simulink model "Motor_Controller"  (R2022a)
settings: Solver=FixedStepDiscrete  StartTime=0.0  StopTime=10.0  FixedStep=Tsi  RelTol=1e-3
values from neighbouring files (symbols this model uses):
  ID_MAP = -123.48613339558477 -123.48613339558477 -123.48613339558477 -123.48613339558477 -44.198759048598419 -53.055770135943519 -71.182249124603388 -83.754050470588808 -83.201735347031459 -88.439458490896953 -101.31743895897192 -109.70740328327217 -114.47442297164962 -116.44804085880824 -116.44444689073586 -115.21087408201925 -125.05741434421833 -119.17821915431119 -119.17821915431119 -119.17821915431119    [PMSM_plant_parameters.sldd]
  IQ_MAP = -339.52155191430609 -339.52155191430609 -339.52155191430609 -339.52155191430609 -298.63834091778995 -232.87622090578927 -192.99576989130705 -164.33367060179748 -138.47181888093323 -120.45650086696185 -110.27189121497848 -100.86088998300514 -91.979080238554033 -83.43921869931269 -75.095588141715126 -66.8406312898249 -66.136785837456742 -332.77622591535993 -332.77622591535993 -332.77622591535993 -33    [PMSM_plant_parameters.sldd]
  Ki_id = 710.3004    [ctrl_parameters.sldd]
  Ki_iq = 1061.5    [ctrl_parameters.sldd]
  Ki_omega = 200.0    [ctrl_parameters.sldd]
  Kp_id = 0.8779    [ctrl_parameters.sldd]
  Kp_iq = 1.0744    [ctrl_parameters.sldd]
  Kp_omega = 3.5    [ctrl_parameters.sldd]
  Ld = 0.00024368    [PMSM_plant_parameters.sldd]
  Lq = 0.00029758    [PMSM_plant_parameters.sldd]
  p = 8.0    [PMSM_plant_parameters.sldd]
  Pmax = 35000.0    [PMSM_plant_parameters.sldd]
  psim = 0.04366    [PMSM_plant_parameters.sldd]
  RPM_VECT = 0.0 500.0 1000.0 1500.0 2000.0 2500.0 3000.0 3500.0 4000.0 4500.0 5000.0 5500.0 6000.0 6500.0 7000.0 7500.0 8000.0    [PMSM_plant_parameters.sldd]
  Tmax = 205.0    [PMSM_plant_parameters.sldd]
  TQ_VECT = -205.0 -200.0 -195.0 -190.0 -185.0 -180.0 -175.0 -170.0 -165.0 -160.0 -155.0 -150.0 -145.0 -140.0 -135.0 -130.0 -125.0 -120.0 -115.0 -110.0 -105.0 -100.0 -95.0 -90.0 -85.0 -80.0 -75.0 -70.0 -65.0 -60.0 -55.0 -50.0 -45.0 -40.0 -35.0 -30.0 -25.0 -20.0 -15.0 -10.0 -5.0 0.0 5.0 10.0 15.0 20.0 25.0 30.0 35.0 40.0 45.0 50.0 55.0 60.0 65.0 70.0 75.0 80.0 85.0 90.0 95.0 100.0 105.0 110.0 115.0 120.0 125.0    [PMSM_plant_parameters.sldd]
  Tsi = 0.0001    [PMSM_system_data.sldd]
  Tso = 0.001    [PMSM_system_data.sldd]
  VDC_VECT = 275.0 300.0 325.0 350.0    [PMSM_plant_parameters.sldd]
  Vnom = 325.0    [PMSM_plant_parameters.sldd]
undefined symbols (not defined in the file or in its folder): denZC_id, denZC_iq, denZC_w, DiscIntNeverNeededParam, ee_sli_rtmsupport, gcbh, numZC_id, numZC_iq, numZC_w
libraries: simulink x8, eeTransforms x2
(part 1 of 2)
settings Model: DataDictionary=PMSM_system_data.sldd  Creator=tshintai  LastModifiedBy=tshintai
settings SolverCC: AlgebraicLoopSolver=TrustRegion
settings DataIOCC: SaveOutput=off  SignalLogging=off  DSMLogging=off  SaveTime=off  ReturnWorkspaceOutputs=off
settings OptimizationCC: DefaultParameterBehavior=Inlined  EnhancedBackFolding=on  PassReuseOutputArgsAs=Individual arguments  ZeroExternalMemoryAtStartup=off  ZeroInternalMemoryAtStartup=off  OptimizeBlockOrder=speed  DifferentSizesBufferReuse=on  OptimizationCustomize=off  EfficientTunableParamExpr=on
settings DebuggingCC: ParameterPrecisionLossMsg=none  ParameterTunabilityLossMsg=error  UnconnectedInputMsg=warning  UnconnectedOutputMsg=warning  UnconnectedLineMsg=warning  SFMachineParentedDataDiag=warning
settings SFSimCC: MATLABDynamicMemAlloc=off
settings RTWCC: SystemTargetFile=ert.tlc  GenCodeOnly=on  TemplateMakefile=ert_default_tmf  GenerateReport=on  IncludeHyperlinkInReport=on  LaunchReport=on  GenerateTraceInfo=on  GenerateTraceReport=on  GenerateTraceReportSl=on  GenerateTraceReportSf=on  GenerateTraceReportEml=on  GenerateCodeMetricsReport=on  DLArmComputeVersion=19.05
settings CodeAppCC: ForceParamTrailComments=on  IgnoreCustomStorageClasses=off  OperatorAnnotations=on  SimulinkDataObjDesc=on  SFDataObjDesc=on  InsertBlockDesc=on
settings ERTTargetCC: TargetLangStandard=C99 (ISO)  GenerateSampleERTMain=on  InlinedParameterPlacement=NonHierarchical  ERTCustomFileTemplate=example_file_process.tlc  EnableUserReplacementTypes=on

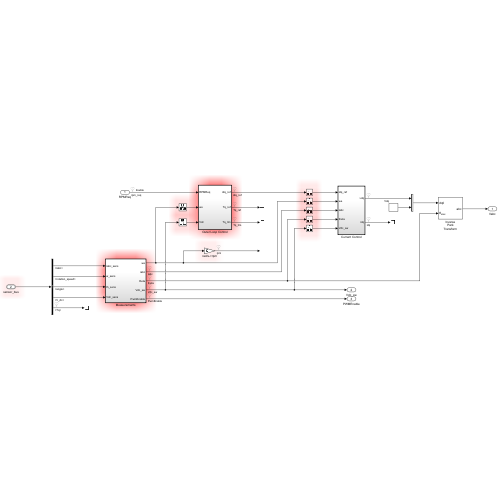
[thumbnail: Simulink's stored preview of the top-level diagram]
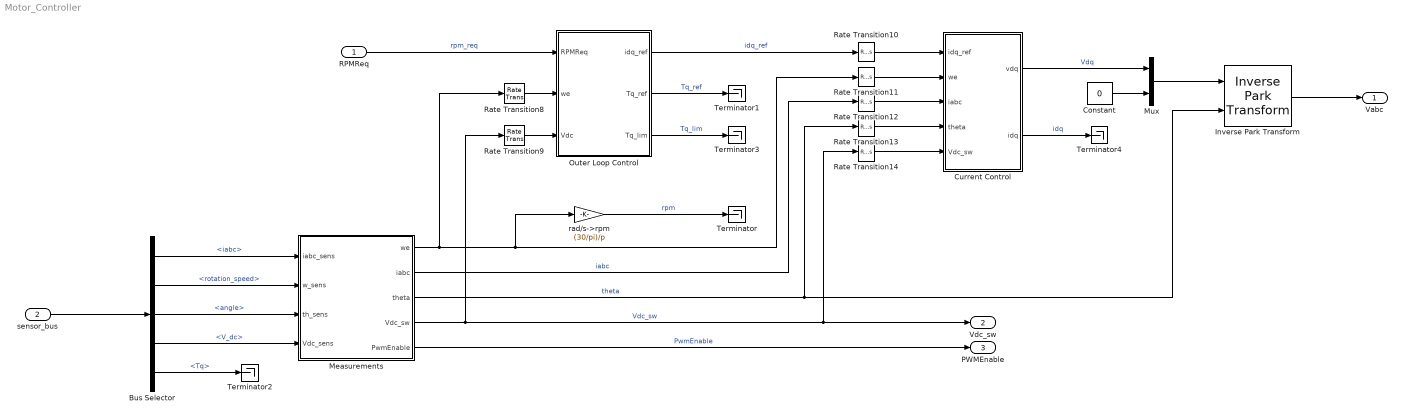
== system Motor_Controller ==
  RPMReq : Inport  OutDataTypeStr=double  PortDimensions=1
  sensor_bus : Inport  Port=2  OutDataTypeStr=Bus: sensor_bus
  Bus Selector : BusSelector  OutputSignals=iabc,rotation_speed,angle,V_dc,Tq
  Constant : Constant  Value=0  OutDataTypeStr=single  SampleTime=-1
  Current Control : Subsystem  TreatAsAtomicUnit=on  SystemSampleTime=1e-4
  Inverse Park Transform : eeTransforms/Inverse Park Transform  AxisAlignment=Q-axis  PowerInvariant=off
  Measurements : Subsystem  TreatAsAtomicUnit=on  SystemSampleTime=Tsi
  Mux : Mux  Inputs=2
  Outer Loop Control : Subsystem  TreatAsAtomicUnit=on  SystemSampleTime=Tso
  Rate Transition{10..14} (5 alike) : RateTransition  OutPortSampleTime=Tsi
  Rate Transition8 : RateTransition  OutPortSampleTime=Tso
  Rate Transition9 : RateTransition  OutPortSampleTime=Tso
  Terminator{,1..4} (5 alike) : Terminator
  rad/s->rpm : Gain  Gain=(30/pi)/p
  Vabc : Outport  VectorParamsAs1DForOutWhenUnconnected=off
  Vdc_sw : Outport  Port=2
  PWMEnable : Outport  Port=3
  wires:
  Rate Transition12/1 -> Current Control/3(iabc)
  Rate Transition13/1 -> Current Control/4(theta)
  Rate Transition14/1 -> Current Control/5(Vdc_sw)
  Bus Selector/1 -> Measurements/1(iabc_sens)  "<iabc>"
  RPMReq/1 -> Outer Loop Control/1(RPMReq)  "rpm_req"
  Bus Selector/2 -> Measurements/2(w_sens)  "<rotation_speed>"
  Mux/1 -> Inverse Park Transform/1
  Measurements/1(we) -> Rate Transition11/1, rad/s->rpm/1, Rate Transition8/1
  Measurements/2(iabc) -> Rate Transition12/1  "iabc"
  Outer Loop Control/1(idq_ref) -> Rate Transition10/1  "idq_ref"
  Current Control/1(vdq) -> Mux/1  "Vdq"
  Current Control/2(idq) -> Terminator4/1  "idq"
  Bus Selector/5 -> Terminator2/1  "<Tq>"
  Measurements/5(PwmEnable) -> PWMEnable/1  "PwmEnable"
  Bus Selector/3 -> Measurements/3(th_sens)  "<angle>"
  Constant/1 -> Mux/2
  Outer Loop Control/3(Tq_lim) -> Terminator3/1  "Tq_lim"
  Rate Transition8/1 -> Outer Loop Control/2(we)
  sensor_bus/1 -> Bus Selector/1
  Bus Selector/4 -> Measurements/4(Vdc_sens)  "<V_dc>"
  Rate Transition10/1 -> Current Control/1(idq_ref)
  Measurements/4(Vdc_sw) -> Vdc_sw/1, Rate Transition14/1, Rate Transition9/1  "Vdc_sw"
  Rate Transition9/1 -> Outer Loop Control/3(Vdc)
  Rate Transition11/1 -> Current Control/2(we)
  Inverse Park Transform/1 -> Vabc/1
  Measurements/3(theta) -> Rate Transition13/1, Inverse Park Transform/2  "theta"
  Outer Loop Control/2(Tq_ref) -> Terminator1/1  "Tq_ref"
  rad/s->rpm/1 -> Terminator/1  "rpm"

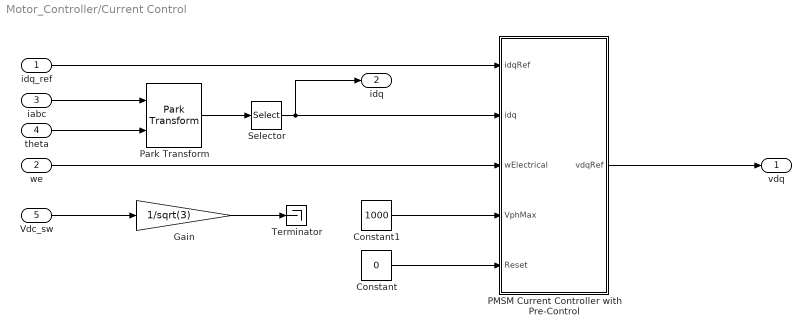
== system Motor_Controller/Current Control ==
  idq_ref : Inport
  we : Inport  Port=2
  iabc : Inport  Port=3
  theta : Inport  Port=4
  Vdc_sw : Inport  Port=5
  Constant : Constant  Value=0  OutDataTypeStr=boolean  SampleTime=-1
  Constant1 : Constant  Value=1000
  Gain : Gain  Gain=1/sqrt(3)
  PMSM Current Controller with Pre-Control : Subsystem  LoadFcn=ee_sli_rtmsupport( 'loadfcn', gcbh );  mask(PMSM Current Controller with Pre-Control){Kp_id=Kp_id, Ki_id=Ki_id, Kaw_id=1, Kp_iq=Kp_iq, Ki_iq=Ki_iq, Kaw_iq=1, Ts=-1, Tsd=Tsi, AxisPrio=Q-axis, ActZC=on, ActFF=on, idVect=[-200, 0, 200], iqVect=[-200, 0, 200], LdMatrix=Ld * ones(3, 3), LqMatrix=Lq * ones(3, 3), psimMatrix=psim * ones(3, 3)}
      mask prompts: Kp_id "physmod:ee:library:comments:control:eePmsmCurrentController:DaxisCurrentProportionalGain_MP"; Ki_id "physmod:ee:library:comments:control:eePmsmCurrentController:DaxisCurrentIntegralGain_MP"; Kaw_id "physmod:ee:library:comments:control:eePmsmCurrentController:DaxisCurrentAntiwindupGain_MP"; Kp_iq "physmod:ee:library:comments:control:eePmsmCurrentController:QaxisCurrentProportionalGain_MP"; Ki_iq "physmod:ee:library:comments:control:eePmsmCurrentController:QaxisCurrentIntegralGain_MP"; Kaw_iq "physmod:ee:library:comments:control:eePmsmCurrentController:QaxisCurrentAntiwindupGain_MP"; Ts "physmod:ee:library:comments:control:eePmsmCurrentController:SampleTime1ForInherited_MP"; Tsd "physmod:ee:library:comments:control:eePmsmCurrentController:DiscretizationSampleTime_MP"; AxisPrio "physmod:ee:library:comments:control:eePmsmCurrentController:AxisPrioritization_MP"; ActZC "physmod:ee:library:comments:control:eePmsmCurrentController:EnableZeroCancellation_MP"; ActFF "physmod:ee:library:comments:control:eePmsmCurrentController:EnablePrecontrolVoltage_MP"; idVect "physmod:ee:library:comments:control:eePmsmCurrentController:DaxisCurrentVectorIdA_MP"; iqVect "physmod:ee:library:comments:control:eePmsmCurrentController:QaxisCurrentVectorIqA_MP"; LdMatrix "physmod:ee:library:comments:control:eePmsmCurrentController:LdMatrixLdidiqH_MP"; LqMatrix "physmod:ee:library:comments:control:eePmsmCurrentController:LqMatrixLqidiqH_MP"; psimMatrix "physmod:ee:library:comments:control:eePmsmCurrentController:PermanentMagnetFluxLinkageMatrixPMidiqWb_MP"
      mask help: physmod:ee:library:comments:control:eePmsmCurrentController:PMSMCurrentControllerWithPreControl_MD
      mask init:
      | [Tsd, numZC_id, denZC_id, numZC_iq, denZC_iq] = ee.mask.initializePmsmCurrentController(ActZC,Ts,Tsd,Kp_id,Ki_id,Kp_iq,Ki_iq);
      | 
      | if length(idVect) < 2            
      | 	error(message('physmod:simscape:compiler:patterns:checks:LengthGreaterThanOrEqual',getString(message('physmod:ee:library:comments:control:eePmsmCurrentController:DaxisCurrentVectorIdA_MP')), '2'));            
      | end
      | if ~all(diff(idVect) > 0)            
      | 	error(message('physmod:simscape:compiler:patterns:checks:StrictlyAscendingVec',getString(message('physmod:ee:library:comments:control:eePmsmCurrentController:DaxisCurrentVectorIdA_MP'))));            
      | end
      | if length(iqVect) < 2            
      | 	error(message('physmod:simscape:compiler:patterns:checks:LengthGreaterThanOrEqual',getString(message('physmod:ee:library:comments:control:eePmsmCurrentController:QaxisCurrentVectorIqA_MP')), '2'));            
      | end
      | if ~all(diff(iqVect) > 0)            
      | 	error(message('physmod:simscape:compiler:patterns:checks:StrictlyAscendingVec',getString(message('physmod:ee:library:comments:control:eePmsmCurrentController:QaxisCurrentVectorIqA_MP'))));            
      | end
      | if ~all(size(LdMatrix) == [length(idVect), length(iqVect)])            
      | 	error(message('physmod:simscape:compiler:patterns:checks:Size2DEqual',getString(message('physmod:ee:library:comments:control:eePmsmCurrentController:LdMatrixLdidiqH_MP')), getString(message('physmod:ee:library:comments:control:eePmsmCurrentController:DaxisCurrentVectorIdA_MP')), getString(message('physmod:ee:library:comments:control:eePmsmCurrentController:QaxisCurrentVectorIqA_MP'))));            
      | end
      | if ~all(size(LqMatrix) == [length(idVect), length(iqVect)])            
      | 	error(message('physmod:simscape:compiler:patterns:checks:Size2DEqual',getString(message('physmod:ee:library:comments:control:eePmsmCurrentController:LqMatrixLqidiqH_MP')), getString(message('physmod:ee:library:comments:control:eePmsmCurrentController:DaxisCurrentVectorIdA_MP')), getString(message('physmod:ee:library:comments:control:eePmsmCurrentController:QaxisCurrentVectorIqA_MP'))));            
      | end
      | if ~all(size(psimMatrix) == [length(idVect), length(iqVect)])            
      | 	error(message('physmod:simscape:compiler:patterns:checks:Size2DEqual',getString(message('physmod:ee:library:comments:control:eePmsmCurrentController:PermanentMagnetFluxLinkageMatrixPMidiqWb_MP')), getString(message('physmod:ee:library:comments:control:eePmsmCurrentController:DaxisCurrentVectorIdA_MP')), getString(message('physmod:ee:library:comments:control:eePmsmCurrentController:QaxisCurrentVectorIqA_MP'))));            
      | end
      settings: CopyFcn=ee_sli_rtmsupport( 'copyfcn', gcbh );  DeleteFcn=ee_sli_rtmsupport( 'deletefcn', gcbh );  ModelCloseFcn=ee_sli_rtmsupport( 'modelclosefcn', gcbh );  PostSaveFcn=ee_sli_rtmsupport( 'postsavefcn', gcbh );  PreCopyFcn=ee_sli_rtmsupport( 'precopyfcn', gcbh );  OpenFcn=ee_sli_rtmsupport( 'openfcn', gcbh );  CloseFcn=ee_sli_rtmsupport( 'closefcn', gcbh );  PreDeleteFcn=ee_sli_rtmsupport( 'predeletefcn', gcbh );
      mask Help: web(nesl_help(gcbh))
      mask Callback Ts: ee.mask.callbackZeroCancellation(gcb);
      mask TypeOptions AxisPrio: d-q Voltage Limiter/AxisPrio
      mask Callback ActZC: ee.mask.callbackZeroCancellation(gcb);
      mask DialogControl Container3 Prompt: physmod:ee:library:comments:control:eePmsmCurrentController:tab_ControlParameters
      mask DialogControl Kp_id Prompt: D 軸電流の比例ゲイン
      mask DialogControl Ki_id Prompt: D 軸電流の積分ゲイン
      mask DialogControl Kaw_id Prompt: D 軸電流のアンチワインドアップ ゲイン
      mask DialogControl Kp_iq Prompt: Q 軸電流の比例ゲイン
      mask DialogControl Ki_iq Prompt: Q 軸電流の積分ゲイン
      mask DialogControl Kaw_iq Prompt: Q 軸電流のアンチワインドアップ ゲイン
      mask DialogControl Ts Prompt: サンプル時間 (継承は -1)
      mask DialogControl Tsd Prompt: 離散化サンプル時間
      mask DialogControl AxisPrio Prompt: 軸の優先順位付け
      mask DialogControl ActZC Prompt: 零点相殺を有効にする
      mask DialogControl ActFF Prompt: プリ制御電圧を有効にする
      mask DialogControl Container4 Prompt: physmod:ee:library:comments:control:eePmsmCurrentController:tab_PreControlParameters
      mask DialogControl idVect Prompt: D 軸電流ベクトル、id (A)
      mask DialogControl iqVect Prompt: Q 軸電流ベクトル、iq (A)
      mask DialogControl LdMatrix Prompt: Ld 行列、Ld(id,iq)、(H)
      mask DialogControl LqMatrix Prompt: Lq 行列、Lq(id,iq)、(H)
      mask DialogControl psimMatrix Prompt: 永久磁石の鎖交磁束の行列、PM(id,iq)、(Wb)
  Park Transform : eeTransforms/Park Transform  AxisAlignment=Q-axis  PowerInvariant=off
  Selector : Selector  InputPortWidth=3  IndexOptions=Index vector (dialog)  Indices=[1 2]  OutputSizes=1
  Terminator : Terminator
  vdq : Outport  VectorParamsAs1DForOutWhenUnconnected=off
  idq : Outport  Port=2  VectorParamsAs1DForOutWhenUnconnected=off
  wires:
  Vdc_sw/1 -> Gain/1
  iabc/1 -> Park Transform/1
  we/1 -> PMSM Current Controller with Pre-Control/3(wElectrical)
  theta/1 -> Park Transform/2
  PMSM Current Controller with Pre-Control/1(vdqRef) -> vdq/1
  idq_ref/1 -> PMSM Current Controller with Pre-Control/1(idqRef)
  Constant/1 -> PMSM Current Controller with Pre-Control/5(Reset)
  Selector/1 -> idq/1, PMSM Current Controller with Pre-Control/2(idq)
  Park Transform/1 -> Selector/1
  Gain/1 -> Terminator/1
  Constant1/1 -> PMSM Current Controller with Pre-Control/4(VphMax)

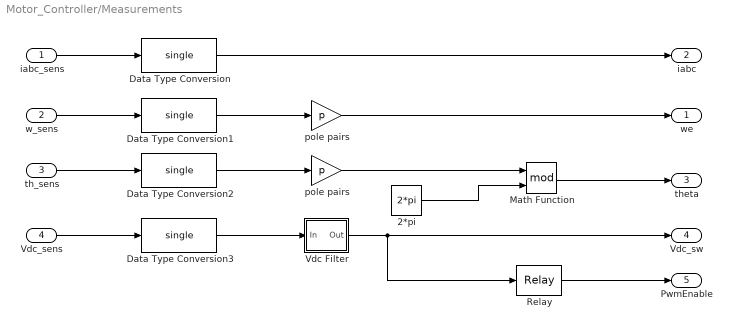
== system Motor_Controller/Measurements ==
  iabc_sens : Inport
  w_sens : Inport  Port=2
  th_sens : Inport  Port=3
  Vdc_sens : Inport  Port=4
  2*pi : Constant  Value=2*pi  OutDataTypeStr=single  SampleTime=-1
  Data Type Conversion{,1..3} (4 alike) : DataTypeConversion  OutDataTypeStr=single  SaturateOnIntegerOverflow=off  RndMeth=Floor
  Math Function : Math  Operator=mod  SignedPower=on
  Relay : Relay  OnSwitchValue=VDC_VECT(1)  OffSwitchValue=0.5*VDC_VECT(1)  OutDataTypeStr=boolean
  Vdc Filter : Subsystem  mask(Discrete first-order filter (Low-pass)){T=0.005, Ts=1e-4}
      mask prompts: T "Time constant (s):"; Ts "Sample time (s):"
      mask help: This block implements a discrete low-pass filter. To calculate the coefficients, the block discretises a continuous low-pass filter using the Tustin method.
      mask init:
      | num = [ Ts/(2*T + Ts), Ts/(2*T + Ts)];
      | den = [ 1, -(2*T - Ts)/(2*T + Ts)];
  pole pairs : Gain  Gain=p
  "pole pairs " : Gain  Gain=p
  we : Outport  VectorParamsAs1DForOutWhenUnconnected=off
  iabc : Outport  Port=2  VectorParamsAs1DForOutWhenUnconnected=off
  theta : Outport  Port=3  VectorParamsAs1DForOutWhenUnconnected=off
  Vdc_sw : Outport  Port=4  VectorParamsAs1DForOutWhenUnconnected=off
  PwmEnable : Outport  Port=5  VectorParamsAs1DForOutWhenUnconnected=off
  wires:
  pole pairs/1 -> we/1
  Vdc_sens/1 -> Data Type Conversion3/1
  th_sens/1 -> Data Type Conversion2/1
  w_sens/1 -> Data Type Conversion1/1
  iabc_sens/1 -> Data Type Conversion/1
  "pole pairs "/1 -> Math Function/1
  2*pi/1 -> Math Function/2
  Math Function/1 -> theta/1
  Relay/1 -> PwmEnable/1
  Vdc Filter/1(Out) -> Relay/1, Vdc_sw/1
  Data Type Conversion/1 -> iabc/1
  Data Type Conversion1/1 -> pole pairs/1
  Data Type Conversion2/1 -> "pole pairs "/1
  Data Type Conversion3/1 -> Vdc Filter/1(In)

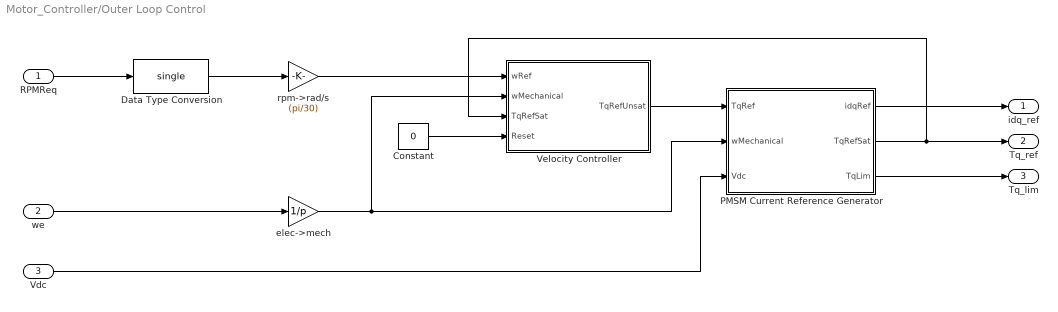
== system Motor_Controller/Outer Loop Control ==
  RPMReq : Inport
  we : Inport  Port=2
  Vdc : Inport  Port=3
  Constant : Constant  Value=0  OutDataTypeStr=boolean  SampleTime=-1
  Data Type Conversion : DataTypeConversion  OutDataTypeStr=single  SaturateOnIntegerOverflow=off  RndMeth=Floor
  PMSM Current Reference Generator : Subsystem  LoadFcn=ee_sli_rtmsupport( 'loadfcn', gcbh );  mask(PMSM Current Reference Generator){Vnom=Vnom, Pmax=Pmax, Tmax=Tmax, Ts=-1, RefType=Lookup-table based, rpmVec=RPM_VECT, TqVec=TQ_VECT, VdcVec=VDC_VECT, PWMMode=SVM: space vector modulation, ModFactor=1, idMatrix=ID_MAP, iqMatrix=IQ_MAP, p=8, psim=0.04, Ld=0.00024, Lq=0.00029, Rs=0.01, RefExpEnable=0}
      mask prompts: Vnom "physmod:ee:library:comments:control:eePmsmCurrentReferenceGen:NominalDclinkVoltageV_MP"; Pmax "physmod:ee:library:comments:control:eePmsmCurrentReferenceGen:MaximumPowerW_MP"; Tmax "physmod:ee:library:comments:control:eePmsmCurrentReferenceGen:MaximumTorqueNm_MP"; Ts "physmod:ee:library:comments:control:eePmsmCurrentReferenceGen:SampleTime1ForInherited_MP"; RefType "physmod:ee:library:comments:control:eePmsmCurrentReferenceGen:CurrentReferences_MP"; rpmVec "physmod:ee:library:comments:control:eePmsmCurrentReferenceGen:MechanicalSpeedVectorWMechanicalrpm_MP"; TqVec "physmod:ee:library:comments:control:eePmsmCurrentReferenceGen:TorqueReferenceVectorTqRefNm_MP"; VdcVec "physmod:ee:library:comments:control:eePmsmCurrentReferenceGen:DClinkVoltageVectorVdcV_MP"; PWMMode "physmod:ee:library:comments:control:eePmsmCurrentReferenceGen:PWMMethod_MP"; ModFactor "physmod:ee:library:comments:control:eePmsmCurrentReferenceGen:ModulationFactor_MP"; idMatrix "physmod:ee:library:comments:control:eePmsmCurrentReferenceGen:DaxisCurrentReferenceMatrixIdwMechanicalTqRefVdcA_MP"; iqMatrix "physmod:ee:library:comments:control:eePmsmCurrentReferenceGen:QaxisCurrentReferenceMatrixIqwMechanicalTqRefVdcA_MP"; p "physmod:ee:library:comments:control:eePmsmCurrentReferenceGen:NumberOfRotorPolePairs_MP"; psim "physmod:ee:library:comments:control:eePmsmCurrentReferenceGen:PermanentMagnetFluxLinkageWb_MP"; Ld "physmod:ee:library:comments:control:eePmsmCurrentReferenceGen:DaxisInductanceH_MP"; Lq "physmod:ee:library:comments:control:eePmsmCurrentReferenceGen:QaxisInductanceH_MP"; Rs "physmod:ee:library:comments:control:eePmsmCurrentReferenceGen:StatorResistanceOhm_MP"; RefExpEnable "physmod:ee:library:comments:control:eePmsmCurrentReferenceGen:ExportCurrentReferences_MP"
      mask help: physmod:ee:library:comments:control:eePmsmCurrentReferenceGen:PMSMCurrentReferenceGenerator_MD
      mask init:
      | if Vnom <= 0            
      |     error(message('physmod:simscape:compiler:patterns:checks:GreaterThanZero',getString(message('physmod:ee:library:comments:control:eePmsmCurrentReferenceGen:NominalDclinkVoltageV_MP'))));            
      | end
      | if Pmax <= 0            
      |     error(message('physmod:simscape:compiler:patterns:checks:GreaterThanZero',getString(message('physmod:ee:library:comments:control:eePmsmCurrentReferenceGen:MaximumPowerW_MP'))));            
      | end
      | if Tmax <= 0            
      |     error(message('physmod:simscape:compiler:patterns:checks:GreaterThanZero',getString(message('physmod:ee:library:comments:control:eePmsmCurrentReferenceGen:MaximumTorqueNm_MP'))));            
      | end
      | switch RefType
      |     case 'Zero d-axis control'
      |         EnableZDAC = 1;
      |         rpmVec = [0, 3000];
      |         TqVec  = [-100, 0, 100];
      |         VdcVec = [300, 350];
      |         idMatrix = zeros(2,3,2);
      |         iqMatrix = zeros(2,3,2);
      |     case 'Lookup-table based'
      |         EnableZDAC = 0;
      |         if length(rpmVec) < 2            
      |             error(message('physmod:simscape:compiler:patterns:checks:LengthGreaterThanOrEqual',getString(message('physmod:ee:library:comments:control:eePmsmCurrentReferenceGen:MechanicalSpeedVectorWMechanicalrpm_MP')), '2'));            
      |         end
      |         if ~all(diff(rpmVec) > 0)            
      |             error(message('physmod:simscape:compiler:patterns:checks:StrictlyAscendingVec',getString(message('physmod:ee:library:comments:control:eePmsmCurrentReferenceGen:MechanicalSpeedVectorWMechanicalrpm_MP'))));            
      |         end
      |         if length(TqVec) < 2            
      |             error(message('physmod:simscape:compiler:patterns:checks:LengthGreaterThanOrEqual',getString(message('physmod:ee:library:comments:control:eePmsmCurrentReferenceGen:TorqueReferenceVectorTqRefNm_MP')), '2'));            
      |         end
      |         if ~all(diff(TqVec) > 0)            
      |             error(message('physmod:simscape:compiler:patterns:checks:StrictlyAscendingVec',getString(message('physmod:ee:library:comments:control:eePmsmCurrentReferenceGen:TorqueReferenceVectorTqRefNm_MP'))));            
      |         end
      |         if length(VdcVec) < 2            
      |             error(message('physmod:simscape:compiler:patterns:checks:LengthGreaterThanOrEqual',getString(message('physmod:ee:library:comments:control:eePmsmCurrentReferenceGen:DClinkVoltageVectorVdcV_MP')), '2'));            
      |         end
      |         if ~all(diff(VdcVec) > 0)            
      |             error(message('physmod:simscape:compiler:patterns:checks:StrictlyAscendingVec',getString(message('physmod:ee:library:comments:control:eePmsmCurrentReferenceGen:DClinkVoltageVectorVdcV_MP'))));            
      |         end
      |         if ~all(size(idMatrix) == [length(rpmVec), length(TqVec), length(VdcVec)])            
      |             error(message('physmod:simscape:compiler:patterns:checks:Size3DEqual',getString(message('physmod:ee:library:comments:control:eePmsmCurrentReferenceGen:DaxisCurrentReferenceMatrixIdwMechanicalTqRefVdcA_MP')), getString(message('physmod:ee:library:comments:control:eePmsmCurrentReferenceGen:MechanicalSpeedVectorWMechanicalrpm_MP')), getString(message('physmod:ee:library:comments:control:eePmsmCurrentReferenceGen:TorqueReferenceVectorTqRefNm_MP')), getString(message('physmod:ee:library:comments:control:eePmsmCurrentReferenceGen:DClinkVoltageVectorVdcV_MP'))));            
      |         end
      |         if ~all(size(iqMatrix) == [length(rpmVec), length(TqVec), length(VdcVec)])            
      |             error(message('physmod:simscape:compiler:patterns:checks:Size3DEqual',getString(message('physmod:ee:library:comments:control:eePmsmCurrentReferenceGen:QaxisCurrentReferenceMatrixIqwMechanicalTqRefVdcA_MP')), getString(message('physmod:ee:library:comments:control:eePmsmCurrentReferenceGen:MechanicalSpeedVectorWMechanicalrpm_MP')), getString(message('physmod:ee:library:comments:control:eePmsmCurrentReferenceGen:TorqueReferenceVectorTqRefNm_MP')), getString(message('physmod:ee:library:comments:control:eePmsmCurrentReferenceGen:DClinkVoltageVectorVdcV_MP'))));            
      |         end
      |     case 'Automatically generated lookup-table'
      |         EnableZDAC = 0;
      |         if Rs <= 0            
      |             error(message('physmod:simscape:compiler:patterns:checks:GreaterThanZero',getString(message('physmod:ee:library:comments:control:eePmsmCurrentReferenceGen:StatorResistanceOhm_MP'))));            
      |         end
      |         if Ld <= 0            
      |             error(message('physmod:simscape:compiler:patterns:checks:GreaterThanZero',getString(message('physmod:ee:library:comments:control:eePmsmCurrentReferenceGen:DaxisInductanceH_MP'))));            
      |         end
      |         if Lq <= 0            
      |             error(message('physmod:simscape:compiler:patterns:checks:GreaterThanZero',getString(message('physmod:ee:library:comments:control:eePmsmCurrentReferenceGen:QaxisInductanceH_MP'))));            
      |         end
      |         
      |         if ModFactor <= 0            
      |             error(message('physmod:simscape:compiler:patterns:checks:GreaterThanZero',getString(message('physmod:ee:library:comments:control:eePmsmCurrentReferenceGen:ModulationFactor_MP'))));            
      |         end
      |         
      |         if ModFactor > 1            
      |             error(message('physmod:simscape:compiler:patterns:checks:LessThanOrEqual',getString(message('physmod:ee:library:comments:control:eePmsmCurrentReferenceGen:ModulationFactor_MP')),'1'));            
      |         end
      |         
      |         % Check if machine parameters were changed
      |         if exist('pmsm_data', 'var')
      |             dataUpdate = (pmsm_data.Ld   ~= Ld)   ||...
      |                          (pmsm_data.Lq   ~= Lq)   ||...
      |                          (pmsm_data.psim ~= psim) ||...
      |                          (pmsm_data.p    ~= p)    ||...
      |                          (pmsm_data.Rs   ~= Rs)   ||...
      |                          (pmsm_data.Pmax ~= Pmax) ||...
      |                          (pmsm_data.Tmax ~= Tmax) ||...
      |                          (pmsm_data.PWMMode ~= PWMMode) ||...
      |                          (pmsm_data.ModFactor ~= ModFactor);
      |         end
      |         % Check if grid points were changed
      |         if exist('grid_points', 'var')
      |             VecUpdate = max(abs(grid_points.RPM_VECT - rpmVec))~=0 ||...
      |                         max(abs(grid_points.TQ_VECT  - TqVec)) ~=0 ||...
      |                         max(abs(grid_points.VDC_VECT - VdcVec))~=0;
      |         end
      |         % Compute current references only IF current references do not exist OR 
      |         % machine parameters were changed OR grid points were changed
      |         if ~exist('pmsm_ref', 'var') || dataUpdate || VecUpdate
      |             grid_points.RPM_VECT = rpmVec;
      |             grid_points.TQ_VECT  = TqVec;
      |             grid_points.VDC_VECT = VdcVec;
      |             pmsm_data.Ld    = Ld; 
      |             pmsm_data.Lq    = Lq; 
      |             pmsm_data.psim  = psim;   
      |             pmsm_data.p     = p;         
      |             pmsm_data.Rs    = Rs;   
      |             pmsm_data.Pmax  = Pmax;      
      |             pmsm_data.Tbase = Tmax;    
      |             pmsm_data.PWMMode   = PWMMode;      
      |             pmsm_data.ModFactor = ModFactor;
      |             pmsm_ref = ee.control.pmsm.getCurrentReferencesPmsm ( pmsm_data, grid_points );
      |             idMatrix = pmsm_ref.idMatrix;
      |             iqMatrix = pmsm_ref.iqMatrix;
      |         end
      |         % Export current references to base workspace
      |         if RefExpEnable==1
      |             assignin('base', 'pmsm_ref', pmsm_ref)
      |             set_param(gcb,'RefExpEnable','0');
      |         end
      | end
      settings: CopyFcn=ee_sli_rtmsupport( 'copyfcn', gcbh );  DeleteFcn=ee_sli_rtmsupport( 'deletefcn', gcbh );  ModelCloseFcn=ee_sli_rtmsupport( 'modelclosefcn', gcbh );  PostSaveFcn=ee_sli_rtmsupport( 'postsavefcn', gcbh );  PreCopyFcn=ee_sli_rtmsupport( 'precopyfcn', gcbh );  OpenFcn=ee_sli_rtmsupport( 'openfcn', gcbh );  CloseFcn=ee_sli_rtmsupport( 'closefcn', gcbh );  PreDeleteFcn=ee_sli_rtmsupport( 'predeletefcn', gcbh );
      mask Help: web(nesl_help(gcbh))
      mask TypeOptions RefType: physmod:ee:library:comments:control:eePmsmCurrentReferenceGen:ZeroD0x2DAxisControl_PV | physmod:ee:library:comments:control:eePmsmCurrentReferenceGen:Lookup0x2DTableBased_PV | physmod:ee:library:comments:control:eePmsmCurrentReferenceGen:AutomaticallyGeneratedLookup0x2DTable_PV
      mask Callback RefType:
      | % Callback function to set the parameters visibility
      | ee.mask.callbackPopupRefGenPmsm(gcb);
      mask TypeOptions PWMMode: physmod:ee:library:comments:control:eePmsmCurrentReferenceGen:SPWMSinusoidalPWM_PV | physmod:ee:library:comments:control:eePmsmCurrentReferenceGen:SVMSpaceVectorModulation_PV
      mask DialogControl Container2 Prompt: physmod:ee:library:comments:control:eePmsmCurrentReferenceGen:tab_GeneralParameters
      mask DialogControl Vnom Prompt: ノミナル DC リンク電圧 (V)
      mask DialogControl Pmax Prompt: 最大出力 (W)
      mask DialogControl Tmax Prompt: 最大トルク (N*m)
      mask DialogControl Ts Prompt: サンプル時間 (継承は -1)
      mask DialogControl Container3 Prompt: physmod:ee:library:comments:control:eePmsmCurrentReferenceGen:tab_ReferenceGenStrategy
      mask DialogControl RefType Prompt: 電流指令値
      mask DialogControl rpmVec Prompt: 機械速度ベクトル、wMechanical (rpm)
      mask DialogControl TqVec Prompt: トルク指令値ベクトル、TqRef (N*m)
      mask DialogControl VdcVec Prompt: DC リンク電圧ベクトル、Vdc (V)
      mask DialogControl PWMMode Prompt: PWM メソッド
      mask DialogControl ModFactor Prompt: 変調係数
      mask DialogControl idMatrix Prompt: D 軸電流の指令値行列、id(wMechanical,TqRef,Vdc)、(A)
      mask DialogControl iqMatrix Prompt: Q 軸電流の指令値行列、iq(wMechanical,TqRef,Vdc)、(A)
      mask DialogControl p Prompt: 回転子極対数
      mask DialogControl psim Prompt: 永久磁石の鎖交磁束 (Wb)
      mask DialogControl Ld Prompt: D 軸インダクタンス (H)
      mask DialogControl Lq Prompt: Q 軸インダクタンス (H)
      mask DialogControl Rs Prompt: 固定子の抵抗 (Ohm)
      mask DialogControl RefExp Prompt: physmod:ee:library:comments:control:eePmsmCurrentReferenceGen:ExportCurrentReferencesToWorkspace_B
      mask DialogControl RefExp Callback:
      | % Enable export of current references
      | set_param(gcb,'RefExpEnable','1');
      mask DialogControl RefExpEnable Prompt: 電流指令値をエクスポート
  Velocity Controller : Subsystem  LoadFcn=ee_sli_rtmsupport( 'loadfcn', gcbh );  mask(Velocity Controller){CtrlType=P-PI control, Kp_w=Kp_omega, Ki_w=Ki_omega, Kv_w=Kp_omega, Kaw_w=100, Ts=-1, Tsd=Tso, ActZC=on}
      mask prompts: CtrlType "physmod:ee:library:comments:control:eeVelocityController:ControlType_MP"; Kp_w "physmod:ee:library:comments:control:eeVelocityController:ControllerProportionalGain_MP"; Ki_w "physmod:ee:library:comments:control:eeVelocityController:ControllerIntegralGain_MP"; Kv_w "physmod:ee:library:comments:control:eeVelocityController:PControllerProportionalGain_MP"; Kaw_w "physmod:ee:library:comments:control:eeVelocityController:IntegralAntiwindupGain_MP"; Ts "physmod:ee:library:comments:control:eeVelocityController:SampleTime1ForInherited_MP"; Tsd "physmod:ee:library:comments:control:eeVelocityController:DiscretizationSampleTime_MP"; ActZC "physmod:ee:library:comments:control:eeVelocityController:EnableZerocancellation_MP"
      mask help: physmod:ee:library:comments:control:eeVelocityController:VelocityController_MD
      mask init:
      | [Ki_w, Kaw_w, Tsd, numZC_w, denZC_w] = ee.mask.initializeVelocityController(CtrlType,Kp_w,Ki_w,Kaw_w,ActZC,Tsd,Ts);
      settings: CopyFcn=ee_sli_rtmsupport( 'copyfcn', gcbh );  DeleteFcn=ee_sli_rtmsupport( 'deletefcn', gcbh );  ModelCloseFcn=ee_sli_rtmsupport( 'modelclosefcn', gcbh );  PostSaveFcn=ee_sli_rtmsupport( 'postsavefcn', gcbh );  PreCopyFcn=ee_sli_rtmsupport( 'precopyfcn', gcbh );  OpenFcn=ee_sli_rtmsupport( 'openfcn', gcbh );  CloseFcn=ee_sli_rtmsupport( 'closefcn', gcbh );  PreDeleteFcn=ee_sli_rtmsupport( 'predeletefcn', gcbh );
      mask Help: web(nesl_help(gcbh))
      mask TypeOptions CtrlType: physmod:ee:library:comments:control:eeVelocityController:PIControl_PV | physmod:ee:library:comments:control:eeVelocityController:PControl_PV | physmod:ee:library:comments:control:eeVelocityController:P0x2DPIControl_PV
      mask Callback CtrlType: ee.mask.callbackPopupVelocityControl(gcb);
      mask Callback Ts: ee.mask.callbackZeroCancellation(gcb);
      mask Callback ActZC: ee.mask.callbackZeroCancellation(gcb);
      mask DialogControl Container1 Prompt: physmod:ee:library:comments:control:eeVelocityController:tab_ControlParameters
      mask DialogControl CtrlType Prompt: コントロール タイプ
      mask DialogControl Kp_w Prompt: コントローラーの比例ゲイン
      mask DialogControl Ki_w Prompt: コントローラーの積分ゲイン
      mask DialogControl Kv_w Prompt: P コントローラーの比例ゲイン
      mask DialogControl Kaw_w Prompt: 積分アンチワインドアップ ゲイン
      mask DialogControl Ts Prompt: サンプル時間 (継承は -1)
      mask DialogControl Tsd Prompt: 離散化サンプル時間
      mask DialogControl ActZC Prompt: 零点相殺を有効にする
  elec->mech : Gain  Gain=1/p
  rpm->rad/s : Gain  Gain=(pi/30)
  idq_ref : Outport  VectorParamsAs1DForOutWhenUnconnected=off
  Tq_ref : Outport  Port=2  VectorParamsAs1DForOutWhenUnconnected=off
  Tq_lim : Outport  Port=3  VectorParamsAs1DForOutWhenUnconnected=off
  wires:
  rpm->rad/s/1 -> Velocity Controller/1(wRef)
  Velocity Controller/1(TqRefUnsat) -> PMSM Current Reference Generator/1(TqRef)
  RPMReq/1 -> Data Type Conversion/1
  we/1 -> elec->mech/1
  Vdc/1 -> PMSM Current Reference Generator/3(Vdc)
  PMSM Current Reference Generator/1(idqRef) -> idq_ref/1
  PMSM Current Reference Generator/2(TqRefSat) -> Tq_ref/1, Velocity Controller/3(TqRefSat)
  PMSM Current Reference Generator/3(TqLim) -> Tq_lim/1
  elec->mech/1 -> PMSM Current Reference Generator/2(wMechanical), Velocity Controller/2(wMechanical)
  Constant/1 -> Velocity Controller/4(Reset)
  Data Type Conversion/1 -> rpm->rad/s/1

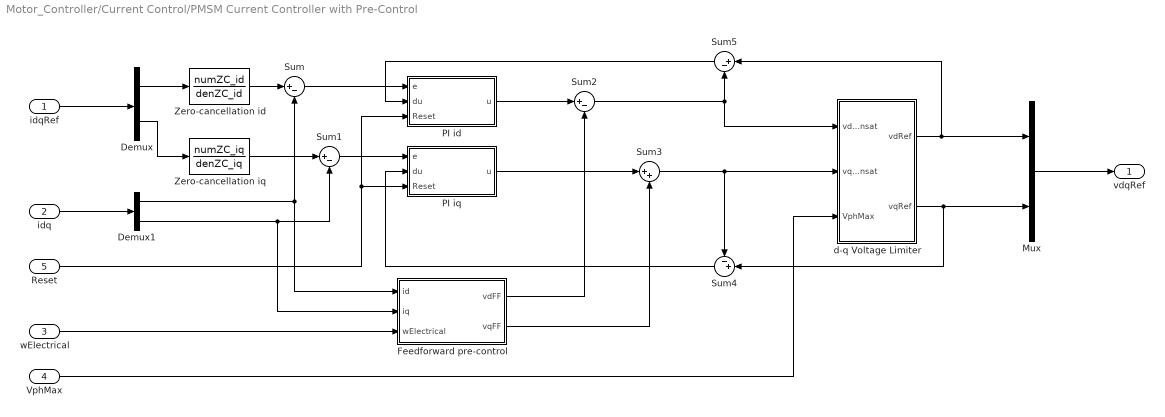
== system Motor_Controller/Current Control/PMSM Current Controller with Pre-Control ==
  idqRef : Inport  SampleTime=Ts
  idq : Inport  Port=2  SampleTime=Ts
  wElectrical : Inport  Port=3  SampleTime=Ts
  VphMax : Inport  Port=4  SampleTime=Ts
  Reset : Inport  Port=5  SampleTime=Ts
  Demux : Demux  Outputs=2
  Demux1 : Demux  Outputs=2
  Feedforward pre-control : Subsystem
  Mux : Mux  Inputs=2
  PI id : Subsystem  LoadFcn=ee_sli_rtmsupport( 'loadfcn', gcbh );  mask(Discrete PI Controller){Kp=Kp_id, Ki=Ki_id, Kaw=Kaw_id, x0=0, Ts=Ts}
      mask prompts: Kp "physmod:ee:library:comments:control:eeDiscretePi:ProportionalGain_MP"; Ki "physmod:ee:library:comments:control:eeDiscretePi:IntegralGain_MP"; Kaw "physmod:ee:library:comments:control:eeDiscretePi:AntiwindupGain_MP"; x0 "physmod:ee:library:comments:control:eeDiscretePi:IntegratorInitialCondition_MP"; Ts "physmod:ee:library:comments:control:eeDiscretePi:SampleTime1ForInherited_MP"
      mask help: physmod:ee:library:comments:control:eeDiscretePi:DiscretePIController_MD
      mask init:
      | if Ts <= 0 && Ts ~= -1            
      |     error(message('physmod:ee:library:MinusOneOrPositive',getString(message('physmod:ee:library:comments:control:eeDiscretePi:SampleTime1ForInherited_MP'))));            
      | end
      settings: CopyFcn=ee_sli_rtmsupport( 'copyfcn', gcbh );  DeleteFcn=ee_sli_rtmsupport( 'deletefcn', gcbh );  ModelCloseFcn=ee_sli_rtmsupport( 'modelclosefcn', gcbh );  PostSaveFcn=ee_sli_rtmsupport( 'postsavefcn', gcbh );  PreCopyFcn=ee_sli_rtmsupport( 'precopyfcn', gcbh );  OpenFcn=ee_sli_rtmsupport( 'openfcn', gcbh );  CloseFcn=ee_sli_rtmsupport( 'closefcn', gcbh );  PreDeleteFcn=ee_sli_rtmsupport( 'predeletefcn', gcbh );
      mask Help: web(nesl_help(gcbh))
      mask DialogControl Container1 Prompt: physmod:ee:library:comments:control:eeDiscretePi:tab_Parameters
      mask DialogControl Kp Prompt: 比例ゲイン
      mask DialogControl Ki Prompt: 積分ゲイン
      mask DialogControl Kaw Prompt: アンチワインドアップ ゲイン
      mask DialogControl x0 Prompt: 積分器の初期条件
      mask DialogControl Ts Prompt: サンプル時間 (継承は -1)
      mask Display: ee.mask.drawDiscretePi(gcb);
  PI iq : Subsystem  LoadFcn=ee_sli_rtmsupport( 'loadfcn', gcbh );  mask(Discrete PI Controller){Kp=Kp_iq, Ki=Ki_iq, Kaw=Kaw_iq, x0=0, Ts=Ts}
      mask prompts: Kp "physmod:ee:library:comments:control:eeDiscretePi:ProportionalGain_MP"; Ki "physmod:ee:library:comments:control:eeDiscretePi:IntegralGain_MP"; Kaw "physmod:ee:library:comments:control:eeDiscretePi:AntiwindupGain_MP"; x0 "physmod:ee:library:comments:control:eeDiscretePi:IntegratorInitialCondition_MP"; Ts "physmod:ee:library:comments:control:eeDiscretePi:SampleTime1ForInherited_MP"
      mask help: physmod:ee:library:comments:control:eeDiscretePi:DiscretePIController_MD
      mask init: same as Motor_Controller/Current Control/PMSM Current Controller with Pre-Control/PI id
      settings: CopyFcn=ee_sli_rtmsupport( 'copyfcn', gcbh );  DeleteFcn=ee_sli_rtmsupport( 'deletefcn', gcbh );  ModelCloseFcn=ee_sli_rtmsupport( 'modelclosefcn', gcbh );  PostSaveFcn=ee_sli_rtmsupport( 'postsavefcn', gcbh );  PreCopyFcn=ee_sli_rtmsupport( 'precopyfcn', gcbh );  OpenFcn=ee_sli_rtmsupport( 'openfcn', gcbh );  CloseFcn=ee_sli_rtmsupport( 'closefcn', gcbh );  PreDeleteFcn=ee_sli_rtmsupport( 'predeletefcn', gcbh );
      mask Help: web(nesl_help(gcbh))
      mask DialogControl Container1 Prompt: physmod:ee:library:comments:control:eeDiscretePi:tab_Parameters
      mask DialogControl Kp Prompt: 比例ゲイン
      mask DialogControl Ki Prompt: 積分ゲイン
      mask DialogControl Kaw Prompt: アンチワインドアップ ゲイン
      mask DialogControl x0 Prompt: 積分器の初期条件
      mask DialogControl Ts Prompt: サンプル時間 (継承は -1)
      mask Display: ee.mask.drawDiscretePi(gcb);
  Sum{,1..2,5} (4 alike) : Sum  Inputs=|+-
  Sum3 : Sum  Inputs=|++
  Sum4 : Sum  Inputs=-+|
  Zero-cancellation id : DiscreteTransferFcn  Numerator=numZC_id  Denominator=denZC_id  SampleTime=Ts
  Zero-cancellation iq : DiscreteTransferFcn  Numerator=numZC_iq  Denominator=denZC_iq  SampleTime=Ts
  d-q Voltage Limiter : Subsystem  LoadFcn=ee_sli_rtmsupport( 'loadfcn', gcbh );  mask(d-q Voltage Limiter){AxisPrio=Q-axis, Ts=Ts}
      mask prompts: AxisPrio "physmod:ee:library:comments:control:eeDqVoltageLimiter:AxisPrioritization_MP"; Ts "physmod:ee:library:comments:control:eeDqVoltageLimiter:SampleTime1ForInherited_MP"
      mask help: physmod:ee:library:comments:control:eeDqVoltageLimiter:dqVoltageLimiter_MD
      settings: CopyFcn=ee_sli_rtmsupport( 'copyfcn', gcbh );  DeleteFcn=ee_sli_rtmsupport( 'deletefcn', gcbh );  ModelCloseFcn=ee_sli_rtmsupport( 'modelclosefcn', gcbh );  PostSaveFcn=ee_sli_rtmsupport( 'postsavefcn', gcbh );  PreCopyFcn=ee_sli_rtmsupport( 'precopyfcn', gcbh );  OpenFcn=ee_sli_rtmsupport( 'openfcn', gcbh );  CloseFcn=ee_sli_rtmsupport( 'closefcn', gcbh );  PreDeleteFcn=ee_sli_rtmsupport( 'predeletefcn', gcbh );
      mask Help: web(nesl_help(gcbh))
      mask TypeOptions AxisPrio: physmod:ee:library:comments:control:eeDqVoltageLimiter:D0x2DAxis_PV | physmod:ee:library:comments:control:eeDqVoltageLimiter:Q0x2DAxis_PV | physmod:ee:library:comments:control:eeDqVoltageLimiter:D0x2DQEquivalence_PV
      mask DialogControl AxisPrio Prompt: 軸の優先順位付け
      mask DialogControl Ts Prompt: サンプル時間 (継承は -1)
  vdqRef : Outport  VectorParamsAs1DForOutWhenUnconnected=off
  wires:
  VphMax/1 -> d-q Voltage Limiter/3(VphMax)
  wElectrical/1 -> Feedforward pre-control/3(wElectrical)
  Reset/1 -> PI id/3(Reset), PI iq/3(Reset)
  idq/1 -> Demux1/1
  idqRef/1 -> Demux/1
  Sum5/1 -> PI id/2(du)
  Demux1/2 -> Sum1/2, Feedforward pre-control/2(iq)
  Demux1/1 -> Sum/2, Feedforward pre-control/1(id)
  d-q Voltage Limiter/2(vqRef) -> Sum4/2, Mux/2
  Sum4/1 -> PI iq/2(du)
  Feedforward pre-control/2(vqFF) -> Sum3/2
  Demux/2 -> Zero-cancellation iq/1
  Sum3/1 -> Sum4/1, d-q Voltage Limiter/2(vqRefUnsat)
  Demux/1 -> Zero-cancellation id/1
  d-q Voltage Limiter/1(vdRef) -> Sum5/1, Mux/1
  Sum/1 -> PI id/1(e)
  Sum1/1 -> PI iq/1(e)
  PI id/1(u) -> Sum2/1
  Zero-cancellation iq/1 -> Sum1/1
  PI iq/1(u) -> Sum3/1
  Mux/1 -> vdqRef/1
  Zero-cancellation id/1 -> Sum/1
  Sum2/1 -> Sum5/2, d-q Voltage Limiter/1(vdRefUnsat)
  Feedforward pre-control/1(vdFF) -> Sum2/2

== system Motor_Controller/Measurements/Vdc Filter ==
  In : Inport
  Discrete Transfer Fcn : DiscreteTransferFcn  Numerator=num  Denominator=den
  Out : Outport  VectorParamsAs1DForOutWhenUnconnected=off
  wires:
  Discrete Transfer Fcn/1 -> Out/1
  In/1 -> Discrete Transfer Fcn/1

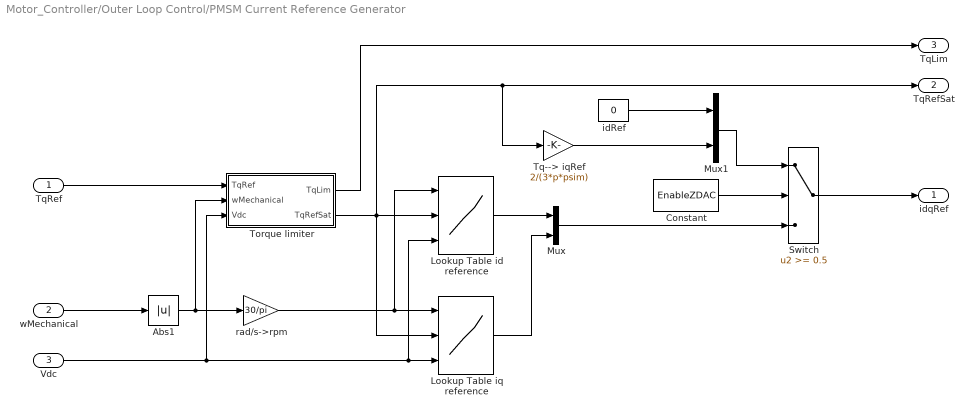
== system Motor_Controller/Outer Loop Control/PMSM Current Reference Generator ==
  TqRef : Inport  SampleTime=Ts
  wMechanical : Inport  Port=2  SampleTime=Ts
  Vdc : Inport  Port=3  SampleTime=Ts
  Abs1 : Abs  SaturateOnIntegerOverflow=off
  Constant : Constant  Value=EnableZDAC  OutDataTypeStr=single  SampleTime=Ts
  Lookup Table id reference : Lookup_n-D  NumberOfTableDimensions=3  BreakpointsForDimension1=rpmVec  BreakpointsForDimension2=TqVec  BreakpointsForDimension3=VdcVec  Table=idMatrix
      settings: InputPortMap=u0,u1,u2
  Lookup Table iq reference : Lookup_n-D  NumberOfTableDimensions=3  BreakpointsForDimension1=rpmVec  BreakpointsForDimension2=TqVec  BreakpointsForDimension3=VdcVec  Table=iqMatrix
      settings: InputPortMap=u0,u1,u2
  Mux : Mux  Inputs=2
  Mux1 : Mux  Inputs=2
  Switch : Switch  Threshold=0.5  SaturateOnIntegerOverflow=off  InputSameDT=off
  Torque limiter : Subsystem
  Tq--> iqRef : Gain  Gain=2/(3*p*psim)
  idRef : Constant  Value=0  OutDataTypeStr=single  SampleTime=Ts
  rad/s->rpm : Gain  Gain=30/pi
  idqRef : Outport  VectorParamsAs1DForOutWhenUnconnected=off
  TqRefSat : Outport  Port=2  VectorParamsAs1DForOutWhenUnconnected=off
  TqLim : Outport  Port=3  VectorParamsAs1DForOutWhenUnconnected=off
  wires:
  Lookup Table id reference/1 -> Mux/1
  Lookup Table iq reference/1 -> Mux/2
  Torque limiter/2(TqRefSat) -> Lookup Table iq reference/2, TqRefSat/1, Tq--> iqRef/1, Lookup Table id reference/2
  Torque limiter/1(TqLim) -> TqLim/1
  rad/s->rpm/1 -> Lookup Table id reference/1, Lookup Table iq reference/1
  Abs1/1 -> Torque limiter/2(wMechanical), rad/s->rpm/1
  Mux1/1 -> Switch/1
  Mux/1 -> Switch/3
  Switch/1 -> idqRef/1
  idRef/1 -> Mux1/1
  Tq--> iqRef/1 -> Mux1/2
  TqRef/1 -> Torque limiter/1(TqRef)
  wMechanical/1 -> Abs1/1
  Vdc/1 -> Lookup Table id reference/3, Lookup Table iq reference/3, Torque limiter/3(Vdc)
  Constant/1 -> Switch/2

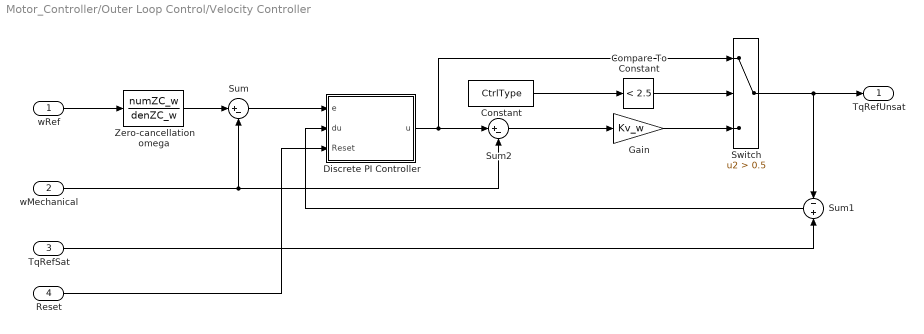
== system Motor_Controller/Outer Loop Control/Velocity Controller ==
  wRef : Inport  SampleTime=Ts
  wMechanical : Inport  Port=2  SampleTime=Ts
  TqRefSat : Inport  Port=3  SampleTime=Ts
  Reset : Inport  Port=4  SampleTime=Ts
  Compare To Constant : simulink/Logic and Bit Operations/Compare To Constant  relop=<  const=2.5  OutDataTypeStr=boolean
  Constant : Constant  Value=CtrlType  OutDataTypeStr=single  SampleTime=Ts
  Discrete PI Controller : Subsystem  LoadFcn=ee_sli_rtmsupport( 'loadfcn', gcbh );  mask(Discrete PI Controller){Kp=Kp_w, Ki=Ki_w, Kaw=Kaw_w, x0=0, Ts=Ts}
      mask prompts: Kp "physmod:ee:library:comments:control:eeDiscretePi:ProportionalGain_MP"; Ki "physmod:ee:library:comments:control:eeDiscretePi:IntegralGain_MP"; Kaw "physmod:ee:library:comments:control:eeDiscretePi:AntiwindupGain_MP"; x0 "physmod:ee:library:comments:control:eeDiscretePi:IntegratorInitialCondition_MP"; Ts "physmod:ee:library:comments:control:eeDiscretePi:SampleTime1ForInherited_MP"
      mask help: physmod:ee:library:comments:control:eeDiscretePi:DiscretePIController_MD
      mask init: same as Motor_Controller/Current Control/PMSM Current Controller with Pre-Control/PI id
      settings: CopyFcn=ee_sli_rtmsupport( 'copyfcn', gcbh );  DeleteFcn=ee_sli_rtmsupport( 'deletefcn', gcbh );  ModelCloseFcn=ee_sli_rtmsupport( 'modelclosefcn', gcbh );  PostSaveFcn=ee_sli_rtmsupport( 'postsavefcn', gcbh );  PreCopyFcn=ee_sli_rtmsupport( 'precopyfcn', gcbh );  OpenFcn=ee_sli_rtmsupport( 'openfcn', gcbh );  CloseFcn=ee_sli_rtmsupport( 'closefcn', gcbh );  PreDeleteFcn=ee_sli_rtmsupport( 'predeletefcn', gcbh );
      mask Help: web(nesl_help(gcbh))
      mask DialogControl Container1 Prompt: physmod:ee:library:comments:control:eeDiscretePi:tab_Parameters
      mask DialogControl Kp Prompt: 比例ゲイン
      mask DialogControl Ki Prompt: 積分ゲイン
      mask DialogControl Kaw Prompt: アンチワインドアップ ゲイン
      mask DialogControl x0 Prompt: 積分器の初期条件
      mask DialogControl Ts Prompt: サンプル時間 (継承は -1)
      mask Display: ee.mask.drawDiscretePi(gcb);
  Gain : Gain  Gain=Kv_w
  Sum : Sum  Inputs=|+-
  Sum1 : Sum  Inputs=-+
  Sum2 : Sum  Inputs=|+-
  Switch : Switch  Criteria=u2 > Threshold  Threshold=0.5  SaturateOnIntegerOverflow=off  InputSameDT=off
  Zero-cancellation omega : DiscreteTransferFcn  Numerator=numZC_w  Denominator=denZC_w  SampleTime=Ts
  TqRefUnsat : Outport  VectorParamsAs1DForOutWhenUnconnected=off
  wires:
  Gain/1 -> Switch/3
  wMechanical/1 -> Sum/2, Sum2/2
  Sum2/1 -> Gain/1
  Sum1/1 -> Discrete PI Controller/2(du)
  wRef/1 -> Zero-cancellation omega/1
  Sum/1 -> Discrete PI Controller/1(e)
  Discrete PI Controller/1(u) -> Sum2/1, Switch/1
  Switch/1 -> TqRefUnsat/1, Sum1/1
  Reset/1 -> Discrete PI Controller/3(Reset)
  Zero-cancellation omega/1 -> Sum/1
  Compare To Constant/1 -> Switch/2
  TqRefSat/1 -> Sum1/2
  Constant/1 -> Compare To Constant/1

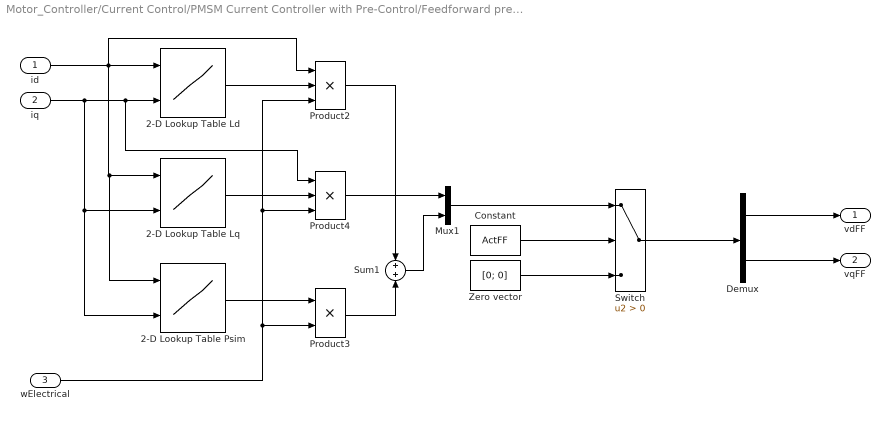
== system Motor_Controller/Current Control/PMSM Current Controller with Pre-Control/Feedforward pre-control ==
  id : Inport
  iq : Inport  Port=2
  wElectrical : Inport  Port=3
  2-D Lookup Table Ld : Lookup_n-D  BreakpointsForDimension1=idVect  BreakpointsForDimension2=iqVect  Table=LdMatrix  ExtrapMethod=Clip  UseLastTableValue=on  InternalRulePriority=Speed  RndMeth=Simplest
      settings: InputPortMap=u0,u1
  2-D Lookup Table Lq : Lookup_n-D  BreakpointsForDimension1=idVect  BreakpointsForDimension2=iqVect  Table=LqMatrix  ExtrapMethod=Clip  InternalRulePriority=Speed  RndMeth=Simplest
      settings: InputPortMap=u0,u1
  2-D Lookup Table Psim : Lookup_n-D  BreakpointsForDimension1=idVect  BreakpointsForDimension2=iqVect  Table=psimMatrix  ExtrapMethod=Clip  InternalRulePriority=Speed  RndMeth=Simplest
      settings: InputPortMap=u0,u1
  Constant : Constant  Value=ActFF  OutDataTypeStr=single  SampleTime=Ts
  Demux : Demux  Outputs=2
  Mux1 : Mux  Inputs=2
  Product2 : Product  Inputs=3
  Product3 : Product
  Product4 : Product  Inputs=3
  Sum1 : Sum
  Switch : Switch  Criteria=u2 > Threshold  SaturateOnIntegerOverflow=off  InputSameDT=off
  Zero vector : Constant  Value=[0; 0]  OutDataTypeStr=single  SampleTime=Ts
  vdFF : Outport  VectorParamsAs1DForOutWhenUnconnected=off
  vqFF : Outport  Port=2  VectorParamsAs1DForOutWhenUnconnected=off
  wires:
  Product2/1 -> Sum1/1
  wElectrical/1 -> Product2/3, Product4/3, Product3/2
  Mux1/1 -> Switch/1
  Product4/1 -> Mux1/1
  id/1 -> 2-D Lookup Table Ld/1, 2-D Lookup Table Lq/1, 2-D Lookup Table Psim/1, Product2/1
  iq/1 -> 2-D Lookup Table Psim/2, 2-D Lookup Table Lq/2, 2-D Lookup Table Ld/2, Product4/1
  2-D Lookup Table Ld/1 -> Product2/2
  Sum1/1 -> Mux1/2
  Zero vector/1 -> Switch/3
  2-D Lookup Table Psim/1 -> Product3/1
  Demux/2 -> vqFF/1
  Demux/1 -> vdFF/1
  Switch/1 -> Demux/1
  Constant/1 -> Switch/2
  2-D Lookup Table Lq/1 -> Product4/2
  Product3/1 -> Sum1/2

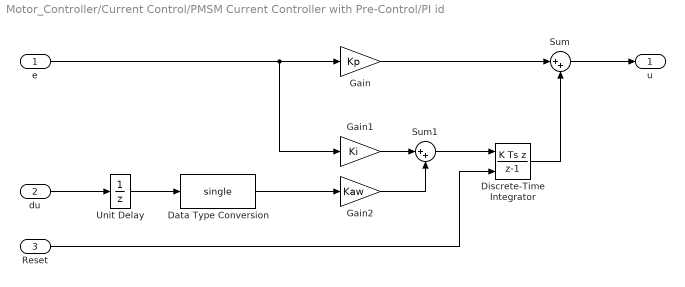
== system Motor_Controller/Current Control/PMSM Current Controller with Pre-Control/PI id ==
  e : Inport  SampleTime=Ts
  du : Inport  Port=2  SampleTime=Ts
  Reset : Inport  Port=3  SampleTime=Ts
  Data Type Conversion : DataTypeConversion  OutDataTypeStr=single  SaturateOnIntegerOverflow=off  RndMeth=Floor
  Discrete-Time Integrator : DiscreteIntegrator  IntegratorMethod=Integration: Backward Euler  ExternalReset=rising  InitialCondition=x0  SampleTime=Ts  ICPrevOutput=DiscIntNeverNeededParam  ICPrevScaledInput=DiscIntNeverNeededParam
  Gain : Gain  Gain=Kp
  Gain1 : Gain  Gain=Ki
  Gain2 : Gain  Gain=Kaw
  Sum : Sum  Inputs=|++
  Sum1 : Sum  Inputs=|++
  Unit Delay : UnitDelay  SampleTime=Ts  HasFrameUpgradeWarning=on
  u : Outport  VectorParamsAs1DForOutWhenUnconnected=off
  wires:
  Unit Delay/1 -> Data Type Conversion/1
  Reset/1 -> Discrete-Time Integrator/2
  du/1 -> Unit Delay/1
  Sum1/1 -> Discrete-Time Integrator/1
  Gain2/1 -> Sum1/2
  e/1 -> Gain1/1, Gain/1
  Gain/1 -> Sum/1
  Gain1/1 -> Sum1/1
  Discrete-Time Integrator/1 -> Sum/2
  Sum/1 -> u/1
  Data Type Conversion/1 -> Gain2/1

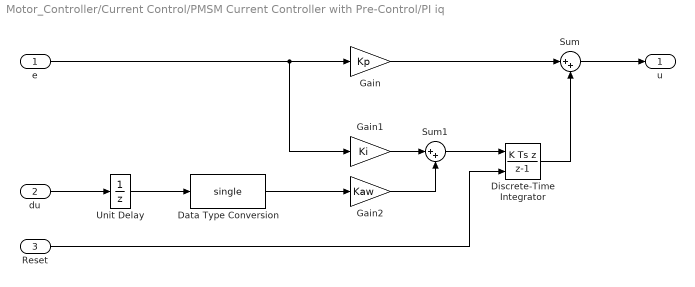
== system Motor_Controller/Current Control/PMSM Current Controller with Pre-Control/PI iq ==
  e : Inport  SampleTime=Ts
  du : Inport  Port=2  SampleTime=Ts
  Reset : Inport  Port=3  SampleTime=Ts
  Data Type Conversion : DataTypeConversion  OutDataTypeStr=single  SaturateOnIntegerOverflow=off  RndMeth=Floor
  Discrete-Time Integrator : DiscreteIntegrator  IntegratorMethod=Integration: Backward Euler  ExternalReset=rising  InitialCondition=x0  SampleTime=Ts  ICPrevOutput=DiscIntNeverNeededParam  ICPrevScaledInput=DiscIntNeverNeededParam
  Gain : Gain  Gain=Kp
  Gain1 : Gain  Gain=Ki
  Gain2 : Gain  Gain=Kaw
  Sum : Sum  Inputs=|++
  Sum1 : Sum  Inputs=|++
  Unit Delay : UnitDelay  SampleTime=Ts  HasFrameUpgradeWarning=on
  u : Outport  VectorParamsAs1DForOutWhenUnconnected=off
  wires:
  Unit Delay/1 -> Data Type Conversion/1
  Reset/1 -> Discrete-Time Integrator/2
  du/1 -> Unit Delay/1
  Sum1/1 -> Discrete-Time Integrator/1
  Gain2/1 -> Sum1/2
  e/1 -> Gain1/1, Gain/1
  Gain/1 -> Sum/1
  Gain1/1 -> Sum1/1
  Discrete-Time Integrator/1 -> Sum/2
  Sum/1 -> u/1
  Data Type Conversion/1 -> Gain2/1
